simulink subsystem "PvtSubSys_VSM_ELK"  (R2020b)
settings: Solver=VariableStepAuto  StartTime=0.0  StopTime=10.0  RelTol=1e-3
values from neighbouring files (symbols this model uses):
  P_VSM_ELK_Curvature_R_Table : value not decoded    [ELK.sldd]
  P_VSM_ELK_Curvature_R_Table_Calibration : value not decoded    [ELK.sldd]
  P_VSM_ELK_Lane_Width_Table : value not decoded    [ELK.sldd]
  P_VSM_ELK_Lane_Width_Table_Calibration : value not decoded    [ELK.sldd]
  P_VSM_ELK_Lateral_Speed_Table : value not decoded    [ELK.sldd]
  P_VSM_ELK_Lateral_Speed_Table_Calibration : value not decoded    [ELK.sldd]
  P_VSM_ELK_OnComing_Lateral = 2.8    [ELK.sldd]
  P_VSM_ELK_OnComing_TTC = 3.0    [ELK.sldd]
  P_VSM_ELK_OverTaking_Lateral = 2.0    [ELK.sldd]
  P_VSM_ELK_OverTaking_TTC = 5.0    [ELK.sldd]
  P_VSM_ELK_Sensitive_Table : value not decoded    [ELK.sldd]
  P_VSM_ELK_Sensitive_Table_Calibration : value not decoded    [ELK.sldd]
  P_VSM_ELK_State_Absesp_enable = 1.0    [ELK.sldd]
  P_VSM_ELK_State_Accpedalrate_enable = 1.0    [ELK.sldd]
  P_VSM_ELK_State_Breakpressure_enable = 1.0    [ELK.sldd]
  P_VSM_ELK_State_DriverInputTrqValue_enable = 1.0    [ELK.sldd]
  P_VSM_ELK_State_Eps_enable = 1.0    [ELK.sldd]
  P_VSM_ELK_State_ESSSts_enable = 1.0    [ELK.sldd]
  P_VSM_ELK_State_Failsafe_enable = 1.0    [ELK.sldd]
  P_VSM_ELK_State_GEAR_enable = 1.0    [ELK.sldd]
  P_VSM_ELK_State_Handson_enable = 1.0    [ELK.sldd]
  P_VSM_ELK_State_Headingangle_enable = 1.0    [ELK.sldd]
  P_VSM_ELK_State_Lane_enable = 1.0    [ELK.sldd]
  P_VSM_ELK_State_LaneChange_enable = 1.0    [ELK.sldd]
  P_VSM_ELK_State_Lanecurve_enable = 1.0    [ELK.sldd]
  P_VSM_ELK_State_LateralAcce_enable = 1.0    [ELK.sldd]
  P_VSM_ELK_State_LongitudeAcc_enable = 1.0    [ELK.sldd]
  P_VSM_ELK_State_Overide_enable = 1.0    [ELK.sldd]
  P_VSM_ELK_State_Param_AngleOffset = 0.05    [ELK.sldd]
  P_VSM_ELK_State_Param_LaneTime : value not decoded    [ELK.sldd]
  P_VSM_ELK_State_Param_Oncoming = 0.55    [ELK.sldd]
  P_VSM_ELK_State_Param_OnTime : value not decoded    [ELK.sldd]
  P_VSM_ELK_State_Param_OutOffset = 0.15    [ELK.sldd]
  P_VSM_ELK_State_Param_Over = 0.55    [ELK.sldd]
  P_VSM_ELK_State_Param_OvTime : value not decoded    [ELK.sldd]
  P_VSM_ELK_State_Param_Speed : value not decoded    [ELK.sldd]
  P_VSM_ELK_State_SteerWheelAngle_enable = 1.0    [ELK.sldd]
  P_VSM_ELK_State_SteerWheelSpd_enable = 1.0    [ELK.sldd]
  P_VSM_ELK_State_TurnLight_enable = 1.0    [ELK.sldd]
  P_VSM_ELK_State_Vehspeed_enable = 1.0    [ELK.sldd]
  P_VSM_ELK_State_Yawsup_enable = 1.0    [ELK.sldd]
undefined symbols (not defined in the file or in its folder): ELKSTATE, P_Global_DxvRearBumper_m, P_Global_IEnvironment_RefPX_Front_Bumper, P_Global_IFV2Fwheel_Dx, P_Global_Vehicle_Length_m, P_Global_VehicleWidthMin_m, P_VSM_LSMC_SampleTime
libraries: simulink x167
(part 2 of 5)

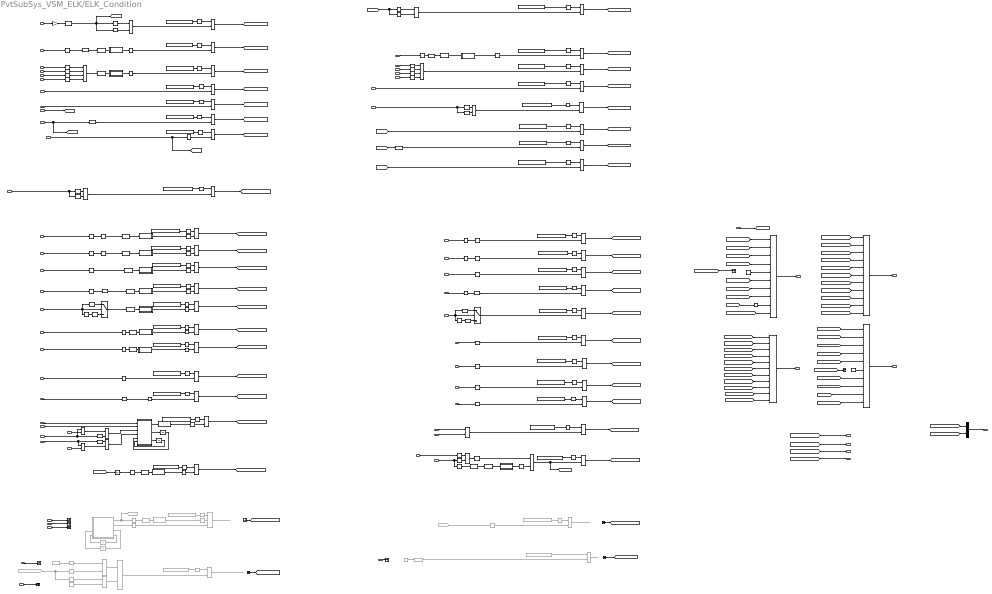
== system PvtSubSys_VSM_ELK/ELK_Condition ==
  note: 后期稳定后，可删除；
      | 1、转向灯条件 标定值/观测量
      | 2、脱手条件 标定值/观测量
      | 20210123
  note: 条件：9
  note: 条件：11
  note: 条件：11
  note: Idle2Ready
      | P_10
  note: 2,3=wrong
  note: 系统当前Selected(Idle)状态非由驾驶员脱手导致
      | ∥由驾驶员脱手导致selected状态需handson
  note: 0x0:Current gear "N" or "P"
      | 0x1:Current gear "1"
      | 0x2:Current gear "2"
      | 0x3:Current gear "3"
      | 0x4:Current gear "4"
      | 0x5:Current gear "5"
      | 0x6:Current gear "6"
      | 0x7:Current gear "7"
      | 0x8:Current gear "R"
      | 0x9-0xF:Reserved
  note: 检测到驾驶员三级脱手报警结束之后
  note: 2,3=wrong
  note: Ready2Idle||Active2Idle
  note: Ready2Active
      | P_10
  note: Active2Ready
  note: OutPut
  note: 此处曾经存在问题
      | override 没有延迟
      | 且double位置存在问题。
  note: 条件：9
  Headingangle_In : Inport
  Headingangle_out : Inport  Port=2
  LaneCurve : Inport  Port=3
  Scene_LaneValid : Inport  Port=4
  LeftChange : Inport  Port=5
  RightChange : Inport  Port=6
  Common_Lane_in : Inport  Port=7
  Common_Lane_Out : Inport  Port=8
  IFC_Failsafe : Inport  Port=9
  ELK_State : Inport  Port=10
  TrqK1 : Inport  Port=11
  canABSVehicleSpd : Inport  Port=12
  canABMVehDynYawRate : Inport  Port=13
  canESPVDCActive : Inport  Port=14
  canESPPTCActive : Inport  Port=15
  canESPBTCActive : Inport  Port=16
  canABSABSActive : Inport  Port=17
  canSASSteerWheelAngle : Inport  Port=18
  canEPSEPS_DriverInputTrqValue : Inport  Port=19
  canSASSteerWheelSpd : Inport  Port=20
  canABMLateralAcce : Inport  Port=21
  LongitudeAcc : Inport  Port=22
  canESP_MasterCylindBrakePress : Inport  Port=23
  canECMAccrPedlPosnDiagc : Inport  Port=24
  canEPSEPS_LKATrqOvlDlvdSts : Inport  Port=25
  CURRENT_GEAR : Inport  Port=26
  canBCMLeftTurnSWSts : Inport  Port=27
  canBCMRightTurnSWSts : Inport  Port=28
  HandsOn : Inport  Port=29
  HandsOffWarnLevel : Inport  Port=30
  HWAActive : Inport  Port=31
  ESSSts : Inport  Port=32
  FLWhelDy : Inport  Port=33
  FRWhelDy : Inport  Port=34
  ActiveZoneIn : Inport  Port=35
  Abs{,1..3,6..8,11,14..16} (11 alike) : Abs
  ActiveZoneIn1 : InportShadow  Port=35
  Bias : Bias  Bias=1.3
  Bus Creator9 : BusCreator  Inputs=2
  CURRENT_GEAR_1 : InportShadow  Port=26
  Compare To Constant{1,12,27,99} (4 alike) : simulink/Logic and Bit Operations/Compare To Constant  Commented=on  relop===  const=0  OutDataTypeStr=boolean
  Compare To Constant{2,4..11,16..18,26,35,40,52,55,81,95,98,105,108,113,121,124} (25 alike) : simulink/Logic and Bit Operations/Compare To Constant  relop===  const=0  OutDataTypeStr=boolean
  Compare To Constant100 : simulink/Logic and Bit Operations/Compare To Constant  relop=<  const=3  OutDataTypeStr=boolean
  Compare To Constant111 : simulink/Logic and Bit Operations/Compare To Constant  relop=>  const=60  OutDataTypeStr=boolean
  Compare To Constant112 : simulink/Logic and Bit Operations/Compare To Constant  relop=<  const=150  OutDataTypeStr=boolean
  Compare To Constant114 : simulink/Logic and Bit Operations/Compare To Constant  relop=>  const=155  OutDataTypeStr=boolean
  Compare To Constant{19,28,32..34,38,41..46,48,50,69,78..79,82,88,115,117..119} (23 alike) : simulink/Logic and Bit Operations/Compare To Constant  relop===  const=1  OutDataTypeStr=boolean
  Compare To Constant116 : simulink/Logic and Bit Operations/Compare To Constant  relop=<  const=55  OutDataTypeStr=boolean
  Compare To Constant{65,72,74,77,94,96,120} (7 alike) : simulink/Logic and Bit Operations/Compare To Constant  relop=>  const=3  OutDataTypeStr=boolean
  Compare To Constant{13,24,47,84,86,90} (6 alike) : simulink/Logic and Bit Operations/Compare To Constant  Commented=on  relop===  const=1  OutDataTypeStr=boolean
  Compare To Constant{14,25,56,92} (4 alike) : simulink/Logic and Bit Operations/Compare To Constant  relop=>  const=1.5  OutDataTypeStr=boolean
  Compare To Constant15 : simulink/Logic and Bit Operations/Compare To Constant  Commented=on  relop=>  const=3  OutDataTypeStr=boolean
  Compare To Constant20 : simulink/Logic and Bit Operations/Compare To Constant  relop=<  const=3  OutDataTypeStr=boolean
  Compare To Constant21 : simulink/Logic and Bit Operations/Compare To Constant  relop===  const=8  OutDataTypeStr=boolean
  Compare To Constant22 : simulink/Logic and Bit Operations/Compare To Constant  relop=<  const=0.2  OutDataTypeStr=boolean
  Compare To Constant23 : simulink/Logic and Bit Operations/Compare To Constant  relop=>  const=1  OutDataTypeStr=boolean
  Compare To Constant29 : simulink/Logic and Bit Operations/Compare To Constant  relop=<  const=70  OutDataTypeStr=boolean
  Compare To Constant3 : simulink/Logic and Bit Operations/Compare To Constant  relop=<  const=2  OutDataTypeStr=boolean
  Compare To Constant30 : simulink/Logic and Bit Operations/Compare To Constant  relop=<  const=2.5  OutDataTypeStr=boolean
  Compare To Constant31 : simulink/Logic and Bit Operations/Compare To Constant  relop=<  const=150  OutDataTypeStr=boolean
  Compare To Constant36 : simulink/Logic and Bit Operations/Compare To Constant  relop=<  const=2  OutDataTypeStr=boolean
  Compare To Constant37 : simulink/Logic and Bit Operations/Compare To Constant  relop=~=  const=4  OutDataTypeStr=boolean
  Compare To Constant39 : simulink/Logic and Bit Operations/Compare To Constant  relop=<  const=2  OutDataTypeStr=boolean
  Compare To Constant49 : simulink/Logic and Bit Operations/Compare To Constant  relop=>  const=0.5  OutDataTypeStr=boolean
  Compare To Constant53 : simulink/Logic and Bit Operations/Compare To Constant  relop=~=  const=5  OutDataTypeStr=boolean
  Compare To Constant54 : simulink/Logic and Bit Operations/Compare To Constant  relop=<  const=0  OutDataTypeStr=boolean
  Compare To Constant57 : simulink/Logic and Bit Operations/Compare To Constant  relop===  const=8  OutDataTypeStr=boolean
  Compare To Constant58 : simulink/Logic and Bit Operations/Compare To Constant  relop=<  const=3  OutDataTypeStr=boolean
  Compare To Constant59 : simulink/Logic and Bit Operations/Compare To Constant  relop=<  const=2.5  OutDataTypeStr=boolean
  Compare To Constant60 : simulink/Logic and Bit Operations/Compare To Constant  relop===  const=5  OutDataTypeStr=boolean
  Compare To Constant61 : simulink/Logic and Bit Operations/Compare To Constant  relop=>  const=90  OutDataTypeStr=boolean
  Compare To Constant62 : simulink/Logic and Bit Operations/Compare To Constant  relop===  const=4  OutDataTypeStr=boolean
  Compare To Constant63 : simulink/Logic and Bit Operations/Compare To Constant  relop=<  const=0.005  OutDataTypeStr=boolean
  Compare To Constant66 : simulink/Logic and Bit Operations/Compare To Constant  relop=>  const=0.6  OutDataTypeStr=boolean
  Compare To Constant67 : simulink/Logic and Bit Operations/Compare To Constant  Commented=on  relop===  const=5  OutDataTypeStr=boolean
  Compare To Constant68 : simulink/Logic and Bit Operations/Compare To Constant  relop=>  const=3.5  OutDataTypeStr=boolean
  Compare To Constant70 : simulink/Logic and Bit Operations/Compare To Constant  relop=>  const=0.25  OutDataTypeStr=boolean
  Compare To Constant71 : simulink/Logic and Bit Operations/Compare To Constant  relop=>  const=5  OutDataTypeStr=boolean
  Compare To Constant73 : simulink/Logic and Bit Operations/Compare To Constant  relop=>  const=200  OutDataTypeStr=boolean
  Compare To Constant75 : simulink/Logic and Bit Operations/Compare To Constant  relop=>  const=3.5  OutDataTypeStr=boolean
  Compare To Constant76 : simulink/Logic and Bit Operations/Compare To Constant  relop=>  const=3.5  OutDataTypeStr=boolean
  Compare To Constant80 : simulink/Logic and Bit Operations/Compare To Constant  relop=>  const=5  OutDataTypeStr=boolean
  Compare To Constant83 : simulink/Logic and Bit Operations/Compare To Constant  relop=>  const=70  OutDataTypeStr=boolean
  Compare To Constant85 : simulink/Logic and Bit Operations/Compare To Constant  relop=>  const=0.006  OutDataTypeStr=boolean
  Compare To Constant89 : simulink/Logic and Bit Operations/Compare To Constant  relop=>  const=1  OutDataTypeStr=boolean
  Compare To Constant91 : simulink/Logic and Bit Operations/Compare To Constant  relop=<  const=30  OutDataTypeStr=boolean
  Constant : Constant  Value=true
  Constant1 : Constant  Value=false
  Data Type Conversion10 : DataTypeConversion  Commented=on  OutDataTypeStr=single
  Data Type Conversion{3..4,6..9,11,14,16..18,27} (12 alike) : DataTypeConversion  OutDataTypeStr=double
  Data Type Conversion2 : DataTypeConversion  Commented=on  OutDataTypeStr=double
  Data Type Conversion5 : DataTypeConversion  Commented=on  OutDataTypeStr=double
  ESSSts1 : InportShadow  Port=32
  From : From  Commented=on  GotoTag=Con_HandOff_Ready2Idle
  From17 : From  Commented=on  GotoTag=Turnlight
  Gain : Gain  Gain=1.03
  Goto33 : Goto  Commented=on  GotoTag=Turnlight
  Ground{,1..3} (4 alike) : Ground
  LeftChange1 : InportShadow  Port=5
  Logical Operator1 : Logic  Inputs=4  AllPortsSameDT=off  OutDataTypeStr=boolean
  Logical Operator{2..3,7,9..12,14,16..19,24,26,38..40,46..48,50,54,57,66} (24 alike) : Logic  AllPortsSameDT=off  OutDataTypeStr=boolean
  Logical Operator13 : Logic  Operator=OR  Inputs=4  AllPortsSameDT=off  OutDataTypeStr=boolean
  Logical Operator{5,15,25,63} (4 alike) : Logic  Commented=on  AllPortsSameDT=off  OutDataTypeStr=boolean
  Logical Operator{4,6,8,20..22,27..34,36..37,49,52..53,64..65,77} (22 alike) : Logic  Operator=OR  AllPortsSameDT=off  OutDataTypeStr=boolean
  Logical Operator23 : Logic  Operator=NOT  AllPortsSameDT=off  OutDataTypeStr=boolean
  Logical Operator35 : Logic  Operator=NOT  AllPortsSameDT=off  OutDataTypeStr=boolean
  Logical Operator41 : Logic  Commented=on  Operator=OR  AllPortsSameDT=off  OutDataTypeStr=boolean
  Logical Operator42 : Logic  Inputs=10  AllPortsSameDT=off  OutDataTypeStr=boolean
  Logical Operator43 : Logic  Operator=OR  Inputs=10  AllPortsSameDT=off  OutDataTypeStr=boolean
  Logical Operator44 : Logic  Inputs=11  AllPortsSameDT=off  OutDataTypeStr=boolean
  Logical Operator45 : Logic  Operator=OR  Inputs=11  AllPortsSameDT=off  OutDataTypeStr=boolean
  Logical Operator51 : Logic  Commented=on  Operator=OR  Inputs=3  AllPortsSameDT=off  OutDataTypeStr=boolean
  Logical Operator58 : Logic  Commented=on  Operator=OR  AllPortsSameDT=off  OutDataTypeStr=boolean
  LongitudeAcc_1 : InportShadow  Port=22
  MATLAB Function : MATLAB Function  TreatAsAtomicUnit=on
  Product : Product
  Relational Operator : RelationalOperator  Operator=>  OutDataTypeStr=boolean  RndMeth=Simplest
  Relational Operator1 : RelationalOperator  Operator=>  OutDataTypeStr=boolean  RndMeth=Simplest
  RightChange1 : InportShadow  Port=6
  Sign : Signum
  Sign1 : Signum
  State_TurnLight2 : MATLAB Function  Commented=on  TreatAsAtomicUnit=on
  Subsystem : Subsystem  mask{Ts=P_VSM_LSMC_SampleTime, Max=10}
      mask prompts: Ts "Sample Time:"; Max "Max Limit:"
      mask Display:
      | Ts=get_param(gcb,'Ts');
      | Max=get_param(gcb,'Max');
      | disp(['Ts:' Ts '\n' 'Max:' Max ]);
  Subsystem1 : Subsystem  mask{Ts=P_VSM_LSMC_SampleTime, Max=10}
      mask prompts: Ts "Sample Time:"; Max "Max Limit:"
      mask Display:
      | Ts=get_param(gcb,'Ts');
      | Max=get_param(gcb,'Max');
      | disp(['Ts:' Ts '\n' 'Max:' Max ]);
  Subsystem10 : Subsystem  mask{Ts=P_VSM_LSMC_SampleTime, Max=10}
      mask prompts: Ts "Sample Time:"; Max "Max Limit:"
      mask Display:
      | Ts=get_param(gcb,'Ts');
      | Max=get_param(gcb,'Max');
      | disp(['Ts:' Ts '\n' 'Max:' Max ]);
  Subsystem11 : Subsystem  mask{Ts=P_VSM_LSMC_SampleTime, Max=10}
      mask prompts: Ts "Sample Time:"; Max "Max Limit:"
      mask Display:
      | Ts=get_param(gcb,'Ts');
      | Max=get_param(gcb,'Max');
      | disp(['Ts:' Ts '\n' 'Max:' Max ]);
  Subsystem12 : Subsystem  mask{Ts=P_VSM_LSMC_SampleTime, Max=10}
      mask prompts: Ts "Sample Time:"; Max "Max Limit:"
      mask Display:
      | Ts=get_param(gcb,'Ts');
      | Max=get_param(gcb,'Max');
      | disp(['Ts:' Ts '\n' 'Max:' Max ]);
  Subsystem15 : Subsystem  mask{Ts=P_VSM_LSMC_SampleTime, Max=10}
      mask prompts: Ts "Sample Time:"; Max "Max Limit:"
      mask Display:
      | Ts=get_param(gcb,'Ts');
      | Max=get_param(gcb,'Max');
      | disp(['Ts:' Ts '\n' 'Max:' Max ]);
  Subsystem17 : Subsystem  mask{Ts=P_VSM_LSMC_SampleTime, Max=10}
      mask prompts: Ts "Sample Time:"; Max "Max Limit:"
      mask Display:
      | Ts=get_param(gcb,'Ts');
      | Max=get_param(gcb,'Max');
      | disp(['Ts:' Ts '\n' 'Max:' Max ]);
  Subsystem2 : Subsystem  Commented=on  mask{Ts=P_VSM_LSMC_SampleTime, Max=10}
      mask prompts: Ts "Sample Time:"; Max "Max Limit:"
      mask Display:
      | Ts=get_param(gcb,'Ts');
      | Max=get_param(gcb,'Max');
      | disp(['Ts:' Ts '\n' 'Max:' Max ]);
  Subsystem4 : Subsystem  mask{Ts=P_VSM_LSMC_SampleTime, Max=10}
      mask prompts: Ts "Sample Time:"; Max "Max Limit:"
      mask Display:
      | Ts=get_param(gcb,'Ts');
      | Max=get_param(gcb,'Max');
      | disp(['Ts:' Ts '\n' 'Max:' Max ]);
  Subsystem5 : Subsystem  mask{Ts=P_VSM_LSMC_SampleTime, Max=10}
      mask prompts: Ts "Sample Time:"; Max "Max Limit:"
      mask Display:
      | Ts=get_param(gcb,'Ts');
      | Max=get_param(gcb,'Max');
      | disp(['Ts:' Ts '\n' 'Max:' Max ]);
  Subsystem6 : Subsystem  mask{Ts=P_VSM_LSMC_SampleTime, Max=10}
      mask prompts: Ts "Sample Time:"; Max "Max Limit:"
      mask Display:
      | Ts=get_param(gcb,'Ts');
      | Max=get_param(gcb,'Max');
      | disp(['Ts:' Ts '\n' 'Max:' Max ]);
  Subsystem7 : Subsystem  mask{Ts=P_VSM_LSMC_SampleTime, Max=10}
      mask prompts: Ts "Sample Time:"; Max "Max Limit:"
      mask Display:
      | Ts=get_param(gcb,'Ts');
      | Max=get_param(gcb,'Max');
      | disp(['Ts:' Ts '\n' 'Max:' Max ]);
  Subsystem8 : Subsystem  mask{Ts=P_VSM_LSMC_SampleTime, Max=10}
      mask prompts: Ts "Sample Time:"; Max "Max Limit:"
      mask Display:
      | Ts=get_param(gcb,'Ts');
      | Max=get_param(gcb,'Max');
      | disp(['Ts:' Ts '\n' 'Max:' Max ]);
  Subsystem9 : Subsystem  mask{Ts=P_VSM_LSMC_SampleTime, Max=10}
      mask prompts: Ts "Sample Time:"; Max "Max Limit:"
      mask Display:
      | Ts=get_param(gcb,'Ts');
      | Max=get_param(gcb,'Max');
      | disp(['Ts:' Ts '\n' 'Max:' Max ]);
  Switch2 : Switch  Criteria=u2 > Threshold
  Switch4 : Switch  Criteria=u2 > Threshold
  Terminator{,1..7} (8 alike) : Terminator
  Unit Delay : UnitDelay  SampleTime=-1  HasFrameUpgradeWarning=on
  Unit Delay1 : UnitDelay  Commented=on  SampleTime=-1  HasFrameUpgradeWarning=on
  Unit Delay4 : UnitDelay  SampleTime=-1  HasFrameUpgradeWarning=on
  Unit Delay5 : UnitDelay  SampleTime=-1  HasFrameUpgradeWarning=on
  Unit Delay8 : UnitDelay  Commented=on  SampleTime=-1  HasFrameUpgradeWarning=on
  canABMLateralAcce_1 : InportShadow  Port=21
  canABMVehDynYawRate_1 : InportShadow  Port=13
  canABSABSActive_1 : InportShadow  Port=17
  canECMAccrPedlPosnDiagc_1 : InportShadow  Port=24
  canEPSEPS_DriverInputTrqValue_1 : InportShadow  Port=19
  canEPSEPS_DriverInputTrqValue_2 : InportShadow  Port=19
  canEPSEPS_LKATrqOvlDlvdSts_1 : InportShadow  Port=25
  canESPBTCActive_1 : InportShadow  Port=16
  canESPPTCActive_1 : InportShadow  Port=15
  canESPVDCActive_1 : InportShadow  Port=14
  canESP_MasterCylindBrakePress_1 : InportShadow  Port=23
  canSASSteerWheelAngle_1 : InportShadow  Port=18
  canSASSteerWheelSpd_1 : InportShadow  Port=20
  param_1 : Constant  Value=P_VSM_ELK_State_Yawsup_enable
  param_10 : Constant  Value=P_VSM_ELK_State_Headingangle_enable
  param_11 : Constant  Value=P_VSM_ELK_State_Failsafe_enable
  param_12 : Constant  Value=P_VSM_ELK_State_Yawsup_enable
  param_13 : Constant  Value=P_VSM_ELK_State_DriverInputTrqValue_enable
  param_14 : Constant  Value=P_VSM_ELK_State_Absesp_enable
  param_15 : Constant  Value=P_VSM_ELK_State_ESSSts_enable
  param_16 : Constant  Value=P_VSM_ELK_State_SteerWheelSpd_enable
  param_17 : Constant  Value=P_VSM_ELK_State_Lanecurve_enable
  param_18 : Constant  Value=P_VSM_ELK_State_LateralAcce_enable
  param_19 : Constant  Value=P_VSM_ELK_State_Eps_enable
  param_2 : Constant  Value=P_VSM_ELK_State_Accpedalrate_enable
  param_20 : Constant  Value=P_VSM_ELK_State_LongitudeAcc_enable
  param_21 : Constant  Value=P_VSM_ELK_State_Accpedalrate_enable
  param_22 : Constant  Commented=on  Value=P_VSM_ELK_State_TurnLight_enable
  param_23 : Constant  Value=P_VSM_ELK_State_GEAR_enable
  param_24 : Constant  Commented=on  Value=P_VSM_ELK_State_TurnLight_enable
  param_25 : Constant  Value=P_VSM_ELK_State_Lane_enable
  param_26 : Constant  Value=P_VSM_ELK_State_Failsafe_enable
  param_27 : Constant  Value=P_VSM_ELK_State_Headingangle_enable
  param_28 : Constant  Value=P_VSM_ELK_State_Breakpressure_enable
  param_29 : Constant  Commented=on  Value=P_VSM_ELK_State_Handson_enable
  param_3 : Constant  Commented=on  Value=P_VSM_ELK_State_Handson_enable
  param_30 : Constant  Value=P_VSM_ELK_State_SteerWheelAngle_enable
  param_31 : Constant  Value=P_VSM_ELK_State_DriverInputTrqValue_enable
  param_32 : Constant  Value=P_VSM_ELK_State_SteerWheelSpd_enable
  param_33 : Constant  Value=P_VSM_ELK_State_LateralAcce_enable
  param_34 : Constant  Value=P_VSM_ELK_State_LongitudeAcc_enable
  param_35 : Constant  Value=P_VSM_ELK_State_Breakpressure_enable
  param_36 : Constant  Value=P_VSM_ELK_State_GEAR_enable
  param_37 : Constant  Value=P_VSM_ELK_State_Overide_enable
  param_38 : Constant  Value=P_VSM_ELK_State_ESSSts_enable
  param_39 : Constant  Value=P_VSM_ELK_State_LaneChange_enable
  param_4 : Constant  Value=P_VSM_ELK_State_Eps_enable
  param_40 : Constant  Value=P_VSM_ELK_State_LaneChange_enable
  param_5 : Constant  Value=P_VSM_ELK_State_Lane_enable
  param_51 : Constant  Value=P_VSM_ELK_State_Overide_enable
  param_52 : Constant  Value=P_VSM_ELK_State_Vehspeed_enable
  param_6 : Constant  Value=P_VSM_ELK_State_SteerWheelAngle_enable
  param_7 : Constant  Value=P_VSM_ELK_State_Lanecurve_enable
  param_8 : Constant  Value=P_VSM_ELK_State_Vehspeed_enable
  param_9 : Constant  Value=P_VSM_ELK_State_Absesp_enable
  ELK_Idle2Ready : Outport
  ELK_Ready2Active : Outport  Port=2
  ELK_Active2Ready : Outport  Port=3
  ELK_Other2Idle : Outport  Port=4
  ELK_TurnLight : Outport  Port=5
  ELK_Con_AccPedalRate_ELKExit : Outport  Port=6
  ELK_Con_BrakePressure_ ELKExit : Outport  Port=7
  ELK_Con_SteerWheelAngle_ ELKExit : Outport  Port=8
  ELK_Con_SteerWheelSpd_ ELKExit : Outport  Port=9
  wires:
  [Con_SteerWheelSpd_Active2Ready] -> ELK_Con_SteerWheelSpd_ ELKExit/1
  [Con_SteerWheelAngle_Active2Ready] -> ELK_Con_SteerWheelAngle_ ELKExit/1
  [Con_BrakePressure_Active2Ready] -> ELK_Con_BrakePressure_ ELKExit/1
  [Con_AccPedalRate_Active2Ready] -> ELK_Con_AccPedalRate_ELKExit/1
  [HWAActive] -> Logical Operator43/9
  Compare To Constant35/1 -> Logical Operator42/9
  [HWAActive] -> Compare To Constant35/1
  HWAActive/1 -> [HWAActive]
  [Con_Override_Ready2Active] -> Logical Operator44/10
  Unit Delay/1 -> Compare To Constant55/1
  Compare To Constant25/1 -> Logical Operator77/2
  param_51/1 -> Compare To Constant81/1
  Compare To Constant55/1 -> Data Type Conversion8/1
  [Overide_condition] -> Unit Delay/1
  Compare To Constant81/1 -> Logical Operator77/1
  Logical Operator77/1 -> [Con_Override_Ready2Active]  "VSM_ELK_Con_Override_Ready2Active"
  Data Type Conversion8/1 -> Subsystem12/1(In1)
  Subsystem12/1(Out1) -> Compare To Constant25/1
  Logical Operator5/1 -> Logical Operator41/2
  Compare To Constant84/1 -> Logical Operator5/2
  Compare To Constant24/1 -> Logical Operator5/1
  [Con_Lane_Idle2Ready] -> Logical Operator42/8
  [Con_VehicleSpeed_Idle2ReadyELK] -> Logical Operator42/7
  Compare To Constant86/1 -> Logical Operator51/3
  State_TurnLight2/2(out) -> Compare To Constant86/1
  Unit Delay8/1 -> State_TurnLight2/4(leftk1)
  State_TurnLight2/3(left) -> Unit Delay8/1
  State_TurnLight2/4(right) -> Unit Delay1/1
  Unit Delay1/1 -> State_TurnLight2/5(rightk1)
  Compare To Constant85/1 -> Logical Operator46/2
  Compare To Constant56/1 -> Data Type Conversion18/1
  canESPBTCActive/1 -> Compare To Constant7/1
  Compare To Constant73/1 -> Logical Operator3/2
  Compare To Constant71/1 -> Logical Operator39/2
  [Con_LaneCurve_Ready2Idle] -> Logical Operator43/4
  Logical Operator14/1 -> [Con_EpsSta_Active2Ready]  "VSM_ELK_Con_EpsSta_Active2Ready"
  canEPSEPS_DriverInputTrqValue_1/1 -> Abs14/1
  Logical Operator34/1 -> [Con_LongitudeAcc_Ready2Active]  "VSM_ELK_Con_LongitudeAcc_Ready2Active"
  Abs16/1 -> Compare To Constant75/1
  Compare To Constant5/1 -> Logical Operator1/1
  canABMVehDynYawRate_1/1 -> Abs6/1
  [Con_EpsSta_Active2Ready] -> Logical Operator45/8
  Logical Operator2/1 -> [Con_DriverInput_Active2Ready]  "VSM_ELK_Con_DriverInput_Active2Ready"
  canSASSteerWheelSpd_1/1 -> Compare To Constant73/1
  canEPSEPS_LKATrqOvlDlvdSts/1 -> Compare To Constant3/1
  Subsystem6/1(Out1) -> Compare To Constant92/1
  Abs11/1 -> Compare To Constant100/1
  Compare To Constant33/1 -> Logical Operator12/1
  [Con_AbsEsp_Ready2Idle] -> Logical Operator43/2
  param_27/1 -> Compare To Constant32/1
  Subsystem4/1(Out1) -> Compare To Constant14/1
  Data Type Conversion2/1 -> Subsystem2/1(In1)
  [Con_SteerWheelSpd_Active2Ready] -> Logical Operator45/3
  Compare To Constant88/1 -> Logical Operator13/3
  canEPSEPS_DriverInputTrqValue/1 -> Abs2/1
  param_35/1 -> Compare To Constant78/1
  Data Type Conversion17/1 -> Subsystem6/1(In1)
  Logical Operator24/1 -> [Con_Failsafe_Ready2Idle]  "VSM_ELK_Con_Failsafe_Ready2Idle"
  Compare To Constant61/1 -> Logical Operator38/2
  Logical Operator40/1 -> [Con_AbsEsp_Ready2Idle]  "VSM_ELK_Con_AbsEsp_Ready2Idle"
  ELK_State/1 -> Terminator5/1
  Compare To Constant59/1 -> Switch2/3
  param_14/1 -> Compare To Constant119/1
  Logical Operator6/1 -> [Con_Headingangel_Idle2Ready]  "VSM_ELK_Con_Headingangel_Idle2Ready"
  Compare To Constant57/1 -> Logical Operator17/2
  param_12/1 -> Compare To Constant118/1
  Abs3/1 -> Compare To Constant56/1
  Compare To Constant27/1 -> Logical Operator51/1
  Compare To Constant29/1 -> Data Type Conversion4/1
  Abs1/1 -> Compare To Constant29/1
  Compare To Constant2/1 -> Logical Operator27/1
  Product/1 -> Compare To Constant54/1
  param_30/1 -> Compare To Constant46/1
  ? -> Compare To Constant67/1
  Compare To Constant1/1 -> Logical Operator58/1
  Compare To Constant21/1 -> Logical Operator35/1
  Compare To Constant65/1 -> Logical Operator27/2
  Common_Lane_Out/1 -> Logical Operator9/2
  Logical Operator63/1 -> ?  "VSM_ELK_Con_HandOff_Ready2Idle"
  canESP_MasterCylindBrakePress_1/1 -> Compare To Constant80/1
  Compare To Constant121/1 -> Logical Operator49/1
  Compare To Constant41/1 -> Logical Operator16/1
  Compare To Constant83/1 -> Logical Operator12/2
  Compare To Constant19/1 -> Logical Operator9/1
  Compare To Constant34/1 -> Logical Operator14/1
  canABSABSActive_1/1 -> Compare To Constant69/1
  [Con_AccPedalRate_Ready2Active] -> Logical Operator44/7
  canESPVDCActive_1/1 -> Compare To Constant79/1
  Logical Operator30/1 -> [Con_AbsEsp_Idle2Ready]  "VSM_ELK_Con_AbsEsp_Idle2Ready"
  param_16/1 -> Compare To Constant8/1
  Compare To Constant76/1 -> Switch4/1
  Compare To Constant95/1 -> Logical Operator29/1
  Compare To Constant3/1 -> Logical Operator33/2
  Logical Operator16/1 -> [Con_OverRide_Active2Ready]  "VSM_ELK_Con_OverRide_Active2Ready"
  param_1/1 -> Compare To Constant95/1
  Compare To Constant43/1 -> Logical Operator7/1
  Abs2/1 -> Compare To Constant30/1
  Subsystem/1(Out1) -> Compare To Constant23/1
  param_10/1 -> Compare To Constant17/1
  Compare To Constant18/1 -> Logical Operator8/1
  State_TurnLight2/1(state) -> Compare To Constant12/1, Goto33/1
  Compare To Constant26/1 -> Logical Operator37/1
  Compare To Constant79/1 -> Logical Operator13/1
  Abs7/1 -> Compare To Constant59/1
  Data Type Conversion18/1 -> Subsystem15/1(In1)
  param_2/1 -> Compare To Constant124/1
  param_32/1 -> Compare To Constant44/1
  [Con_CURRENT_GEAR_Active2Ready] -> Logical Operator45/10
  param_26/1 -> Compare To Constant28/1
  Data Type Conversion3/1 -> Subsystem7/1(In1)
  canSASSteerWheelSpd/1 -> Compare To Constant31/1
  canBCMRightTurnSWSts/1 -> Terminator4/1
  Compare To Constant77/1 -> Switch4/3
  [Con_AccPedalRate_Active2Ready] -> Logical Operator45/7
  Compare To Constant47/1 -> Logical Operator15/1
  param_4/1 -> Compare To Constant105/1
  param_3/1 -> Compare To Constant1/1
  Compare To Constant8/1 -> Logical Operator31/1
  Logical Operator37/1 -> [Con_CURRENT_GEAR_Ready2Active]  "VSM_ELK_Con_CURRENT_GEAR_Ready2Active"
  Data Type Conversion14/1 -> Subsystem11/1(In1)
  Subsystem2/1(Out1) -> Compare To Constant15/1
  [Con_HandOff_Ready2Idle] -> Terminator1/1
  [Con_LateralAcc_Active2Ready] -> Logical Operator45/4
  canABMLateralAcce/1 -> Abs11/1
  canABSVehicleSpd/1 -> Gain/1
  Compare To Constant58/1 -> Switch2/1
  Compare To Constant13/1 -> Logical Operator15/2
  param_11/1 -> Compare To Constant18/1
  Sign/1 -> Product/1
  Compare To Constant14/1 -> Logical Operator52/2
  CURRENT_GEAR_1/1 -> Compare To Constant57/1
  [Con_CURRENT_GEAR_Ready2Active] -> Logical Operator44/9
  param_28/1 -> Compare To Constant121/1
  Logical Operator28/1 -> [Con_DriverInput_Ready2Active]  "VSM_ELK_Con_DriverInput_Ready2Active"
  From17/1 -> Compare To Constant13/1
  Compare To Constant66/1 -> Logical Operator47/2
  param_18/1 -> Compare To Constant9/1
  Logical Operator11/1 -> [Con_BrakePressure_Active2Ready]  "VSM_ELK_Con_BrakePressure_Active2Ready"
  param_33/1 -> Compare To Constant43/1
  Logical Operator17/1 -> [Con_CURRENT_GEAR_Active2Ready]  "VSM_ELK_Con_CURRENT_GEAR_Active2Ready"
  canEPSEPS_LKATrqOvlDlvdSts_1/1 -> Compare To Constant89/1
  param_21/1 -> Compare To Constant33/1
  param_20/1 -> Compare To Constant11/1
  Logical Operator27/1 -> [Con_SteerWheelAngle_Ready2Active]  "VSM_ELK_Con_SteerWheelAngle_Ready2Active"
  Sign1/1 -> Product/2
  Compare To Constant124/1 -> Logical Operator52/1
  param_19/1 -> Compare To Constant34/1
  Logical Operator47/1 -> Logical Operator16/2, [Overide_condition]
  Gain/1 -> Bias/1
  [Headingangle] -> Logical Operator26/2
  Subsystem7/1(Out1) -> Compare To Constant94/1
  Compare To Constant99/1 -> Logical Operator25/2
  Logical Operator12/1 -> [Con_AccPedalRate_Active2Ready]  "VSM_ELK_Con_AccPedalRate_Active2Ready"
  [Con_BrakePressure_Active2Ready] -> Logical Operator45/6
  Logical Operator39/1 -> [Con_YawRate_Ready2Idle]  "VSM_ELK_Con_YawRate_Ready2Idle"
  IFC_Failsafe/1 -> [IFC_Failsafe], Logical Operator23/1
  Subsystem15/1(Out1) -> Compare To Constant66/1
  LongitudeAcc_1/1 -> Switch4/2, Compare To Constant76/1, Abs15/1
  canABMLateralAcce_1/1 -> Abs16/1
  Compare To Constant90/1 -> Logical Operator25/1
  Logical Operator42/1 -> ELK_Idle2Ready/1  "VSM_ELK_Idle2Ready"
  Logical Operator57/1 -> Logical Operator64/2
  Compare To Constant91/1 -> Data Type Conversion7/1
  [Con_EpsSta_Ready2Active] -> Logical Operator44/8
  Compare To Constant48/1 -> Logical Operator17/1
  Compare To Constant75/1 -> Logical Operator7/2
  Compare To Constant116/1 -> Logical Operator65/1
  Logical Operator32/1 -> [Con_LateralAcc_Ready2Active]  "VSM_ELK_Con_LateralAcc_Ready2Active"
  Abs14/1 -> Compare To Constant68/1
  Data Type Conversion27/1 -> Subsystem5/1(In1)
  Logical Operator33/1 -> [Con_EpsSta_Ready2Active]  "VSM_ELK_Con_EpsSta_Ready2Active"
  canEPSEPS_DriverInputTrqValue_2/1 -> Abs3/1, Sign1/1
  Compare To Constant67/1 -> Data Type Conversion5/1
  Logical Operator65/1 -> Logical Operator66/2
  Compare To Constant42/1 -> Logical Operator10/1
  Logical Operator64/1 -> [Con_VehicleSpeed_Idle2ReadyELK]  "VSM_ELK_Con_VehicleSpeed_Idle2ReadyELK"
  Compare To Constant92/1 -> Logical Operator49/2
  Scene_LaneValid/1 -> Terminator2/1
  Switch2/1 -> Data Type Conversion3/1
  [Con_LongitudeAcc_Ready2Active] -> Logical Operator44/5
  [Con_BrakePressure_Ready2Active] -> Logical Operator44/6
  Compare To Constant72/1 -> Logical Operator28/2
  [Con_Failsafe_Ready2Idle] -> Logical Operator43/3
  Compare To Constant96/1 -> Logical Operator32/2
  [IFC_Failsafe] -> Logical Operator24/2
  [Con_SteerWheelAngle_Active2Ready] -> Logical Operator45/1
  Compare To Constant11/1 -> Logical Operator34/1
  [Con_SteerWheelAngle_Ready2Active] -> Logical Operator44/1
  Logical Operator58/1 -> ?  "VSM_ELK_Con_Handson_Idle2Ready"
  [Con_SteerWheelSpd_Ready2Active] -> Logical Operator44/3
  param_25/1 -> Compare To Constant19/1
  Compare To Constant120/1 -> Logical Operator30/2
  Abs15/1 -> Compare To Constant77/1
  Compare To Constant80/1 -> Logical Operator11/2
  [Con_DriverInput_Ready2Active] -> Logical Operator44/2
  canESPVDCActive/1 -> Compare To Constant5/1
  [Con_LaneCurve_Idle2Ready] -> Logical Operator42/6
  param_34/1 -> Compare To Constant42/1
  Compare To Constant115/1 -> Logical Operator46/1
  Logical Operator49/1 -> [Con_BrakePressure_Ready2Active]  "VSM_ELK_Con_BrakePressure_Ready2Active"
  Logical Operator38/1 -> [Con_SteerWheelAngle_Active2Ready]  "VSM_ELK_Con_SteerWheelAngle_Active2Ready"
  Compare To Constant28/1 -> Logical Operator24/1
  Compare To Constant15/1 -> Logical Operator51/2
  Logical Operator4/1 -> [Con_Lane_Idle2Ready]  "VSM_ELK_Con_Lane_Idle2Ready"
  Compare To Constant100/1 -> Data Type Conversion14/1
  From/1 -> Compare To Constant99/1, Compare To Constant24/1
  Compare To Constant17/1 -> Logical Operator6/1
  Data Type Conversion7/1 -> Subsystem4/1(In1)
  Logical Operator29/1 -> [Con_YawRate_Idle2Ready]  "VSM_ELK_Con_YawRate_Idle2Ready"
  canESP_MasterCylindBrakePress/1 -> Compare To Constant20/1
  Compare To Constant4/1 -> Logical Operator28/1
  Compare To Constant23/1 -> Logical Operator29/2
  Logical Operator8/1 -> [Con_Failsafe_Idle2Ready]  "VSM_ELK_Con_Failsafe_Idle2Ready"
  Compare To Constant89/1 -> Logical Operator14/2
  param_6/1 -> Compare To Constant2/1
  [Con_Headingangle_Ready2Idle] -> Logical Operator43/5
  Logical Operator25/1 -> Logical Operator41/1
  Data Type Conversion10/1 -> Compare To Constant90/1
  Compare To Constant108/1 -> Logical Operator36/1
  Abs/1 -> Compare To Constant22/1
  Logical Operator7/1 -> [Con_LateralAcc_Active2Ready]  "VSM_ELK_Con_LateralAcc_Active2Ready"
  [Con_LongitudeAcc_Active2Ready] -> Logical Operator45/5
  Data Type Conversion6/1 -> Subsystem9/1(In1)
  Subsystem11/1(Out1) -> Compare To Constant96/1
  Logical Operator10/1 -> [Con_LongitudeAcc_Active2Ready]  "VSM_ELK_Con_LongitudeAcc_Active2Ready"
  CURRENT_GEAR/1 -> Compare To Constant21/1
  Compare To Constant70/1 -> Data Type Conversion27/1
  Common_Lane_in/1 -> Logical Operator4/2
  Compare To Constant117/1 -> Logical Operator66/1
  Compare To Constant114/1 -> Logical Operator65/2
  [Con_DriverInput_Active2Ready] -> Logical Operator45/2
  Compare To Constant105/1 -> Logical Operator33/1
  Compare To Constant98/1 -> Logical Operator30/1
  Compare To Constant12/1 -> Data Type Conversion2/1
  [Con_OverRide_Active2Ready] -> Logical Operator45/9
  Logical Operator43/1 -> ELK_Other2Idle/1  "VSM_ELK_Other2Idle"
  param_8/1 -> Compare To Constant117/1
  Headingangle_out/1 -> [Headingangle]
  canABSABSActive/1 -> Compare To Constant10/1
  param_13/1 -> Compare To Constant4/1
  canABMVehDynYawRate/1 -> Abs/1
  param_17/1 -> Compare To Constant115/1
  Compare To Constant111/1 -> Logical Operator57/1
  canESPBTCActive_1/1 -> Compare To Constant88/1
  Compare To Constant113/1 -> Logical Operator64/1
  Logical Operator3/1 -> [Con_SteerWheelSpd_Active2Ready]  "VSM_ELK_Con_SteerWheelSpd_Active2Ready"
  Logical Operator35/1 -> Logical Operator37/2
  Data Type Conversion11/1 -> Subsystem10/1(In1)
  param_9/1 -> Compare To Constant98/1
  Data Type Conversion4/1 -> Subsystem8/1(In1)
  canESPPTCActive_1/1 -> Compare To Constant82/1
  param_52/1 -> Compare To Constant113/1
  Compare To Constant112/1 -> Logical Operator57/2
  HandsOn/1 -> Terminator6/1
  Compare To Constant94/1 -> Logical Operator34/2
  Compare To Constant82/1 -> Logical Operator13/2
  [Con_TurnLight_Active2Ready] -> Bus Creator9/2
  param_29/1 -> Logical Operator63/1
  canECMAccrPedlPosnDiagc_1/1 -> Compare To Constant83/1
  Logical Operator52/1 -> [Con_AccPedalRate_Ready2Active]  "VSM_ELK_Con_AccPedalRate_Ready2Active"
  Compare To Constant69/1 -> Logical Operator13/4
  LaneCurve/1 -> [LaneCurve], Compare To Constant63/1
  Compare To Constant74/1 -> Logical Operator31/2
  canSASSteerWheelAngle_1/1 -> Abs8/1
  Headingangle_In/1 -> Logical Operator6/2
  param_36/1 -> Compare To Constant48/1
  [Con_VehicleSpeed_Ready2IdleELK] -> Logical Operator43/7
  Logical Operator31/1 -> [Con_SteerWheelSpd_Ready2Active]  "VSM_ELK_Con_SteerWheelSpd_Ready2Active"
  Compare To Constant78/1 -> Logical Operator11/1
  Logical Operator45/1 -> ELK_Active2Ready/1  "VSM_ELK_Active2Ready"
  [Con_AbsEsp_Idle2Ready] -> Logical Operator42/2
  param_22/1 -> Compare To Constant47/1
  param_37/1 -> Compare To Constant41/1
  Logical Operator46/1 -> [Con_LaneCurve_Ready2Idle]  "VSM_ELK_Con_LaneCurve_Ready2Idle"
  Subsystem10/1(Out1) -> Compare To Constant74/1
  [Con_Lane_Ready2Idle] -> Logical Operator43/8
  Bus Creator9/1 -> ELK_TurnLight/1  "ELK_TurnLight"
  [Con_YawRate_Idle2Ready] -> Logical Operator42/1
  Logical Operator1/1 -> Data Type Conversion9/1
  Logical Operator26/1 -> [Con_Headingangle_Ready2Idle]  "VSM_ELK_Con_Headingangle_Ready2Idle"
  Logical Operator66/1 -> [Con_VehicleSpeed_Ready2IdleELK]  "VSM_ELK_Con_VehicleSpeed_Ready2Idle"
  param_5/1 -> Compare To Constant16/1
  Compare To Constant68/1 -> Logical Operator2/2
  Switch4/1 -> Logical Operator10/2
  canECMAccrPedlPosnDiagc/1 -> Compare To Constant91/1
  Compare To Constant118/1 -> Logical Operator39/1
  Logical Operator13/1 -> Logical Operator40/2  "absespsup"
  param_7/1 -> Compare To Constant108/1
  [LaneCurve] -> Compare To Constant85/1
  canSASSteerWheelAngle/1 -> Abs1/1
  canESPPTCActive/1 -> Compare To Constant6/1
  Compare To Constant16/1 -> Logical Operator4/1
  param_23/1 -> Compare To Constant26/1
  Logical Operator36/1 -> [Con_LaneCurve_Idle2Ready]  "VSM_ELK_Con_LaneCurve_Idle2Ready"
  Compare To Constant32/1 -> Logical Operator26/1
  Compare To Constant9/1 -> Logical Operator32/1
  [Con_YawRate_Ready2Idle] -> Logical Operator43/1
  Compare To Constant20/1 -> Data Type Conversion17/1
  canBCMLeftTurnSWSts/1 -> Terminator3/1
  LongitudeAcc/1 -> Abs7/1, Compare To Constant58/1, Switch2/2
  [Con_Handson_Idle2Ready] -> Terminator/1
  param_24/1 -> Compare To Constant27/1
  [Con_Headingangel_Idle2Ready] -> Logical Operator42/3
  Logical Operator41/1 -> Logical Operator58/2
  Compare To Constant63/1 -> Logical Operator36/2
  Logical Operator51/1 -> ?  "VSM_ELK_Con_TurnLight_Ready2Active"
  Subsystem17/1(Out1) -> Compare To Constant120/1
  Abs8/1 -> Compare To Constant61/1
  Logical Operator44/1 -> ELK_Ready2Active/1  "VSM_ELK_Ready2Active"
  Logical Operator23/1 -> Logical Operator8/2
  [Con_LateralAcc_Ready2Active] -> Logical Operator44/4
  Subsystem5/1(Out1) -> Compare To Constant71/1
  Compare To Constant46/1 -> Logical Operator38/1
  Compare To Constant6/1 -> Logical Operator1/2
  Compare To Constant30/1 -> Data Type Conversion6/1
  Compare To Constant31/1 -> Data Type Conversion11/1
  [Con_Failsafe_Idle2Ready] -> Logical Operator42/4
  Data Type Conversion16/1 -> Subsystem/1(In1)
  Bias/1 -> [speed], Compare To Constant112/1, Compare To Constant111/1
  Logical Operator9/1 -> [Con_Lane_Ready2Idle]  "VSM_ELK_Con_Lane_Ready2Idle"
  Compare To Constant45/1 -> Logical Operator2/1
  Compare To Constant7/1 -> Logical Operator1/3
  Compare To Constant119/1 -> Logical Operator40/1
  [Con_TurnLight_Ready2Active] -> Bus Creator9/1
  Compare To Constant44/1 -> Logical Operator3/1
  Subsystem9/1(Out1) -> Compare To Constant72/1
  Logical Operator15/1 -> ?  "VSM_ELK_Con_TurnLight_Active2Ready"
  Compare To Constant10/1 -> Logical Operator1/4
  Abs6/1 -> Compare To Constant70/1
  Compare To Constant54/1 -> Logical Operator47/1
  TrqK1/1 -> Sign/1
  Compare To Constant22/1 -> Data Type Conversion16/1
  Subsystem8/1(Out1) -> Compare To Constant65/1
  [speed] -> Compare To Constant114/1, Compare To Constant116/1
  Data Type Conversion5/1 -> Logical Operator63/2
  param_31/1 -> Compare To Constant45/1
  Data Type Conversion9/1 -> Subsystem17/1(In1)
  Compare To Constant52/1 -> Logical Operator22/1
  Compare To Constant53/1 -> Logical Operator18/2
  Logical Operator18/1 -> Logical Operator22/2
  Compare To Constant37/1 -> Logical Operator18/1
  param_15/1 -> Compare To Constant52/1
  ESSSts/1 -> Compare To Constant53/1, Compare To Constant37/1
  Logical Operator22/1 -> [Con_ESSSts_Idle2Ready]  "VSM_ELK_Con_ESSSts_Idle2Ready"
  [Con_ESSSts_Idle2Ready] -> Logical Operator42/10
  [Con_ESSSts_Ready2Idle] -> Logical Operator43/10
  Compare To Constant60/1 -> Logical Operator20/2
  Compare To Constant38/1 -> Logical Operator19/1
  Compare To Constant62/1 -> Logical Operator20/1
  Logical Operator19/1 -> [Con_ESSSts_Ready2Idle]  "VSM_ELK_Con_ESSSts_Ready2Idle"
  Logical Operator20/1 -> Logical Operator19/2
  ESSSts1/1 -> Compare To Constant62/1, Compare To Constant60/1
  param_38/1 -> Compare To Constant38/1
  Relational Operator1/1 -> Logical Operator48/1
  ActiveZoneIn/1 -> Relational Operator1/2
  Logical Operator50/1 -> MATLAB Function/4(Rdy)  "LKA_Rdy"
  Relational Operator/1 -> Logical Operator50/2
  Compare To Constant36/1 -> Logical Operator48/2
  ActiveZoneIn1/1 -> Relational Operator/2
  MATLAB Function/3(Rfg) -> Unit Delay5/1
  Compare To Constant39/1 -> Logical Operator50/1
  Logical Operator48/1 -> MATLAB Function/3(Ldy)  "LKA_Ldy"
  Unit Delay4/1 -> MATLAB Function/5(Lfgk1)
  Compare To Constant49/1 -> Logical Operator21/2
  RightChange/1 -> MATLAB Function/2(RightChangefg)
  MATLAB Function/1(y) -> Subsystem1/1(In1)
  Unit Delay5/1 -> MATLAB Function/6(Rfgk1)
  Subsystem1/1(Out1) -> Compare To Constant49/1
  LeftChange/1 -> MATLAB Function/1(LeftChangefg)
  MATLAB Function/2(Lfg) -> Unit Delay4/1
  param_39/1 -> Compare To Constant40/1
  Logical Operator21/1 -> [Con_LaneChange_Ready2Active]  "VSM_ELK_Con_LaneChange_Ready2Active"
  FLWhelDy/1 -> Relational Operator1/1, Compare To Constant36/1
  Compare To Constant40/1 -> Logical Operator21/1
  FRWhelDy/1 -> Compare To Constant39/1, Relational Operator/1
  [Con_LaneChange_Ready2Active] -> Logical Operator44/11
  param_40/1 -> Compare To Constant50/1
  Logical Operator54/1 -> [Con_LaneChange_Active2Ready]  "VSM_ELK_Con_LaneChange_Active2Ready"
  LeftChange1/1 -> Logical Operator53/1
  RightChange1/1 -> Logical Operator53/2
  Compare To Constant50/1 -> Logical Operator54/1
  Logical Operator53/1 -> Logical Operator54/2
  [Con_LaneChange_Active2Ready] -> Logical Operator45/11
  Constant/1 -> Logical Operator42/5
  Constant1/1 -> Logical Operator43/6
  Ground/1 -> [Con_TurnLight_Ready2Active]
  Ground1/1 -> [Con_Handson_Idle2Ready]
  HandsOffWarnLevel/1 -> Terminator7/1
  Ground2/1 -> [Con_TurnLight_Active2Ready]
  Ground3/1 -> [Con_HandOff_Ready2Idle]
